simulink model "Study_1"  (R2023b)
settings: Solver=ode23s  StartTime=0.0  StopTime=150  RelTol=1e-3
values from neighbouring files (symbols this model uses):
  B = 1    [Study_1_data.m]
  K = 1    [Study_1_data.m]
  Kg = 0.8    [Study_1_data.m]
  M = 1    [Study_1_data.m]
  s = tf('s')    [Study_1_data.m]
libraries: slctrl_linear x15, simulink x6
settings Model: Creator=user  LastModifiedBy=user
settings SolverCC: AlgebraicLoopSolver=TrustRegion
settings DebuggingCC: UnconnectedInputMsg=warning  UnconnectedOutputMsg=warning  UnconnectedLineMsg=warning
settings ModelReferenceCC: EnableRefExpFcnMdlSchedulingChecks=on
settings RTWCC: DLArmComputeVersion=19.05

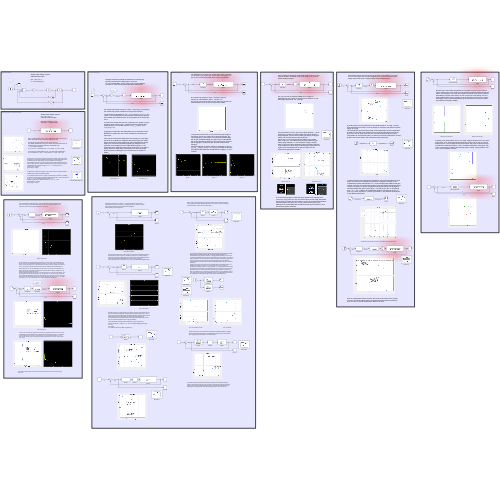
[thumbnail: Simulink's stored preview of the top-level diagram]
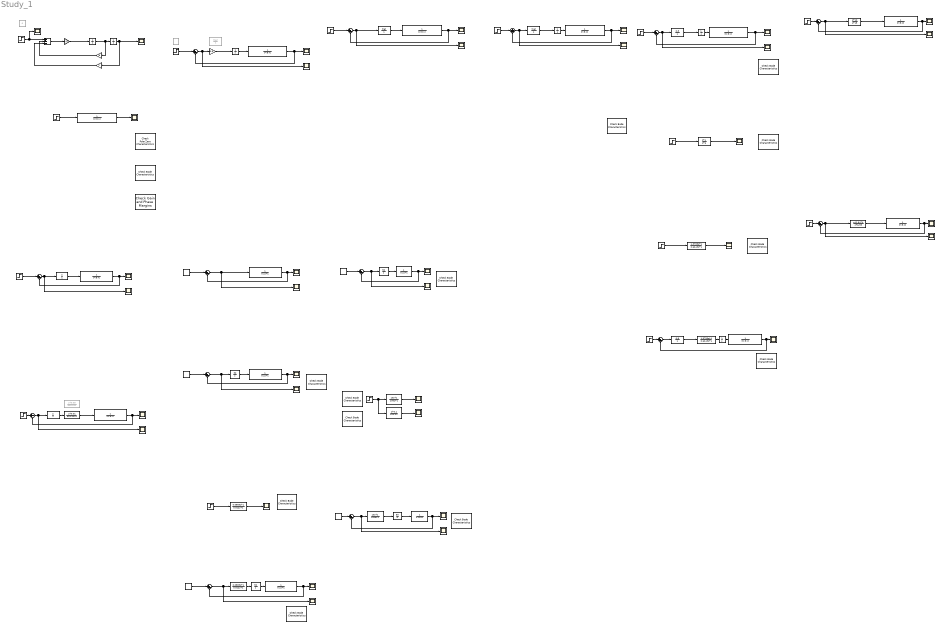
== system Study_1 ==
  note: Root Locus Study
  note: Closed loop System
  note: Basic Analysis for 2nd order system
  note: Differential Model
  note: @ Kg = 1
  note: Further more, we can plot our system response for frequency spectrum using
      | bode plots, by previous knowlegde we know that a second order system acts
      | as a filter due to its inertial nature, this is illustrated in the bode plot.
      | Quick bode plot preview, our second order system causes a decrease in gain after certain frequency, called the cutoff frequency, phase and gain margin are caulcated also from a bode plot, @ m = b = k = 1, cutoff freq at w = 1,
      | phase margin = 90 deg
      | gain margin = infinity.
  note: This is a second order system, using suitable calculations we can get certain parameters from it (rise time, settling time, etc)
      |
      | first lets get the pole locations for the open loop plant:
      | from simple calculations for this plant, there are 2 poles which have an imaginary part, the poles are found by characteristic eqn : (-b+- root(b^2-4ac))/2a
      | for m = b = k = 1, poles are at s1 = -0.5 + 0.86j , s2 = -0.5 - 0.86j
      |
      | we can find our natural frequency wn , and zeta from standard form
      | s^2 + 2*zeta*wn*s + wn^2 , in our case wn = 1 rad/s , zeta = 0.5
  note: Simple mass damper system
      | differential Eq model
      |
      | mx'' + bx' + kx = f
      | x'' = (F-kx-bx')(1/m)
  note: Simple mass damper system
      | mx'' + bx' + kx = F
      | Transfer function model
      |
      | (ms^2+bs+k)*X(s) = F(s)
      | X(s)/F(s) = 1/(ms^2+bs+k)
  note: studying closed loop systems is essential for controlling our plant and choosing the suitable type of controller.
      | For our demonstration, we are going to use a unity feedback controller, ie. Ideal sensing with no transient charactertics.
  note: the closed loop transfer function is: Gcl(s) = G(s)*Gc(s)/(1+G(s)Gc(s))
      | this closed loop system is stable from the previous analysis.
      |
      | The final value is calculated by, lim s->0 (1/s) *s*Gcl(s) = (1)/(1+1) = 0.5 ,where 1/s is the step input, s is from the final value theorem, and Gcl is the closed loop transfer function, so this system has an overall gain of 0.5
      |
      | to observe the steady state error for a step input, our system is a type 0 system, while a step is type 1, meaning that there will be a finite steady state error, to calculate the error -> lim s->0 s.R(s)/1+G(s) = 1/(1+(1/1)) = 0.5
  note: to assess our closed loop behavior even more we can do a nyquist plot to find stability margins and overall stability status.
      |
      | in our default example we have 2 open loop poles which 0 of them is unstable, and from the plot we have 0 clockwise rotations around the -1 point, from the rule: Z = N + P , -> the unstable closed loop poles are 0.
      | Stability margins for the default numbers of m = b = k = 1, are:
      | Phase margin = 90 deg
      | Gain margin = infinity
  note: by applying a ramp input, the steady state error is infinity due to the difference in system type, this can be illustrated by connecting the ramp input.
      |
      | if we want to eliminate the steady state error entirely for a step input, we can do so by adding an integrator (pole at the origin) this makes the input type equal to the system type, which eliminates the steady state error, this can be illustrated by adding an integrator block,
      | (note that: if the integrator block is added while the gain is 1, the system becomes marginally stable, which doesnt allow us to see the steady state error elimination, for illustration, we removed the Kg block and put a constant gain of 0.5 to make sure the system is stable.)
  note: Lets study the root locus for our closed loop system, assuming our controller is just a gain, lets see the effect of changing our gain on our closed loop system poles location and stability.
  note: Our closed loop system is: Gcl(s) = K*G(s)/(1+G(s)*K)
      | therefore our characteristic eqn is: 1+G(s)*K = 0,
      | lets plot our root locus for this c/cs eqn, this can't be done from inside simulink but we can do this from within matlab
  note: From the shown root locus we can see that the gain margin is sure infinite, and for our system as we increase the gain, the natural frequency of the system is increased and the damping ratio is also increased making the system more underdamped, this can be illustrated by observing the system's step response after changing the controller's gain, also the steady state is changing.
      | A general approach for steady state error assuming the gain is Kg, lim s->0 s.R(s)/(1+G(s)) = 1/(1+(Kg/1)), therefore we see that increasing Kg decreases the steady state error (@Kg = 5, Ess = 0.16667)
  note: @ Kg = 5
  note: @ Kg = 30
  note: Lets try adding an integrator to eliminate steady state error, then observe the effect of adding a pole at the origin on our overall system stability margins.
  note: Our c/cs eqn has an integrator added so we expect an additional pole, the number of asymptotes increases to 3, and their angles become 60, -60, 180 deg.
  note: From the shown root locus, we can see that if the gain > 1, then we become unstable, the system totally changed by adding a single integrator, it went from an infinite gain margin to tiny gain margin, we can illustrate this using bode plots.
      | Put our Kg = 0.5, this causes the gain margin to be 6.02db which is gain of 2, this makes sense since the maximum gain before going unstable is 1, also the phase margin is 50 deg which is fine as the larger the phase margin the faster response of the system, this can be seen by observing the settling time for a gain of 0.5 and settling time for gain of 0.8 (this can be achieved using stepinfo in matlab)
  note: Bode for Kg = 0.5
  note: Output @ Kg = 0.5
  note: Error @ Kg = 0.5
  note: Bode for Kg = 0.8
  note: As we increased the gain to make the poles approach the imaginary axis even more, ie: Kg from 0.5 to 0.8, we notice that the phase margin decreased, meaning that the system became harder to control as the phase shift between input and output is too large, also, as the system comes closer to the imaginary axis, the damping ratio decreases and the system settles in more time and has greater overshoot
  note: Lets assume that the system we have is the worst case possible, a Kg value of 0.8, it has 2 poles very near the imaginary axis, and it has almost no gain margin (we put the Kg as 0.8 permanently in the controller block)
  note: by observing the current system we have a phase margin of 14.3 deg , Lets put some requirements to meet, in order to design out controller, lets assume a phase margin of 30 deg.
      | This requirement can be achieved using a lead compensator, a lead compensator is made of a zero and a pole where the zero comes at lower frequency than the pole, ie the zero is closer to the real axis, this causes the bode plot of a lead compensator to have positive phase, so when we put a lead compensator, we add phase to the current system, this is illustrates using a bode plot.
  note: In order to find the lead compensator parameters, we should calculate how much phase we need, for our example we need about 16 degrees of phase, so our compensator's phase shift should be 16 + 6 (the 6 degrees are added as the gain shift will cause the zero-crossover frequency to be also shifted reducing the phase margin once again), to get the compensator equation that achieves 22 degrees maximum phase shift, get a (for 22 deg a = 2.2) and tao (for Wm =1.08 rad/s @ gain = -3.4 , tao = 0.6243), the compensator equation becomes ((a*tao*s)+1)/((tao*s)+1) which equates to (1.3735s+1)/(0.6243s+1), lets observe the bode plot of the added compensator.
  note: Another way to use a lead compensator is if we want to move our root locus to meet a certain point on the s plane, this is possible because by adding a pole and a zero, and the pole is to the left, this causes the centroid of the loci to be shifted left making the system more stable, we can control how much shifting occurs to meet a specific pole location, allowing us to get accurate results from our system, the shifting in the loci is illustrated below (for this illustration we used the system G(s) without an integrator added)
  note: Without lead compensator
  note: With lead compensator
  note: Currently our 2 poles location are at -0.5+-0.86j, suppose we want our lous to pass by the point -2+2j, using the angle argument (for a point to be on the loic, sum of angles of poles - sum of angles of zeros must equal 180), from the below analysis we find that to meet this condition, 145+113+thetaPole-thetaZero must equal 180, I chose a zero angle of 100deg, then the pole angle is 22deg, using geometry: zero is at -1.6474, and pole is at-6.95
  note: Compensator adds 22 deg at frequency of 0.88rad/s and also adds 3.43 db
  note: And our compensator doesnt work-ish, this is due to the nature of the system we have, its critically stable that any small gain increase causes our phase to drop so much, so a lead compensator doesn't work here.
  note: If our system has a steady state error, a lag compensator can be designed to limit that error using the root locus method, assume we have the system below, it has a SS error of 0.33 using a gain controller with value of 2.
  note: from the equation Z/P = (Gd(0)-Ess*Gd(0))/(Ess.Gn(0)), we can choose our desired Ess and get the ratio for our lag compensator transfer function, where Z is the location of the zero and P is the location of the pole, noting that for a lag compensator, the pole corner freq is always lower than the zero, so on the s-plane the pole will be to the left of the zero (opposite to a lead compensator).
      |
      | Assume an Ess of 0.1, then by substituting in the eqn: Z/P = 4.5, to create our compensator, we need to choose the zero position, First thing to know, we dont want to affect our original loci in the s-plane we just want to eliminate SS error.
      | The angle argument theorem tells us that for a point to fall on the loci, the sum of pole angles - sum of zero angles to that point must equal 180, so to not affect this loci, the pole and zero must be as close to each other as possible, so to the far right near the orgin, a good rule of thumb is to take the zero location as the Re(Dominant pole)/50, for our example our dominant pole is at s = -0.5+ 0.86j, so the zero is at s = -0.01, and the pole is at s=-0.0022, lets add our compensator.
  note: Before compensator
  note: From the root locus and error graphs we can see that our compensator works, the root locus and our dominant poles aren't affected, and the steady state error decreases to reach 0.1, the problem is that the reponse time is too slow, it takes about 10 mins to reach the desired error, so if we move the pole and zero a bit to the left the repsonse should be faster (let zero be -0.05 and pole be at -0.011)
  note: After compensator
  note: The response time got faster as the zero and pole were shifted to the left, but the rootlocus got bent more.
  note: Lets assume a plant of tf = 1/(0.2s+1) -> first order system, we have some requirements to meet in this system, a steady state error of less than 0.02 for ramp input and phase margin of greater than 48 degrees.
      | Lets first study our existing system.
  note: From analysis and from the existing graph, we can see that the steady state error is infinite, as the system type is 0, and the input type is 2, by adding a pole at origin to the system the steady state error can be finite, and by adding a gain we can choose our desired steady state error, Ess = R(s)/(1+(KG(s))).
      | so we calculate our K to be 50 for an error of 0.02, so we add an integrator (50/s)
  note: Error before Integrator
  note: Error after Integrator
  note: Now lets move to our phase margin reuqirements, from the bode plot we can see that we have about 18 degrees of phase margin and infinite gain margin, so we have a requirement of adding about 30 degrees of phase, this requirement can be achieved using a lead compensator, but also a lag compensator, a lag compensator can be used to solve both requirements at the same time, we will first use a lead compensator then the lag compensator.
      |
      | using calculations to design lead compensator: (a*tao*s+1)/(tao*s+1)
      | assume we add 30 + 7 degrees = 37 , W = 22 rad after adding gain1/root(a)
      | a = 4.02
      | tao = 0.022
      | our equation becomes (0.0885+1)/(0.022*s+1)
  note: We can use a lag compensator to achieve the phase margin required, he idea is that by shifting the whole magnitude plot down, we move the crossover frequency to lower frequency giving us more phase margin,
  note: by looking at the bode plot we see that to achieve a phase margin of 48 we need to shift the plot by subtracting about 18.5 db lets approximate to 20db, for a compensator to give gain shift of 20db, -> 20log(k)=20db, therefore k=10, then our compensator equation becomes (tao*s+1)/(beta*tao*s+1) where beta is 10, unlike a lead compensator we don't need to care about the phase shift of this compensator or at what frequency it's put, simply we choose a low frequency to not affect the dominant poles, and make sure the shift is totally applied before the zero crossover frequency.
      | a good rule of thumb is to choose the zero location at the dominantpole/50, in our equation this is Szero= -5/50 = -0.1, then the pole is at -0.1/10 = 0.01, our compensator equation becomes: (10*s+1)/(100*s+1) , note that the equation should be written like this because we are subtracting gain from 0 (at low freq s=jw=0, eqn evaluates to gain of 1 while at high freq s=jw=inf, eqn evaluates to 1/10,but if we write our equation as (s+0.1)/(s+0.01)), at low freq s=jw=0, eqn evaluates to gain of 1/10, while at freq s=jw=inf, eqn evaluates to gain of 1, we want the first case since we subtract gain from the total system, this is further illustrated below)
  note: This is the behavior we want
  note: This is undesired
  note: We can see that our compensator decreases gain by 20db and applies a negative phase shift of about 55deg at freq of 0.032rad/s, this should also be visible below when applying the compensator on the whole system.
  note: As we can see from the plot above the phase margin was increased to 50.5deg, and the gain crossover frequency was moved to 4 rad/s (previous analysis showed that the new crossover freq would be 4.43 rad/s), the spike at 0.0306 rad is due to applying the lag compensator which decreases phase at a chosen frequency
  Add : Sum  Inputs=+--
  Bode Plot : slctrl_linear/Check Bode  Characteristics  InstantiateOnLoad=on  SaveOperatingPoints=off  LinearizationIOs={'/Step1', 1, 'in', 'on', '';'/Transfer Fcn', 1, 'out', 'on', ''}  LinearizeAt=SnapshotTimes  SnapshotTimes=[0]  TriggerType=rising  SampleTime=auto  RateConversionMethod=zoh  PreWarpFreq=10  UseExactDelayModel=off  UseFullBlockNameLabels=off  UseBusSignalLabels=off  enabled=on  stopWhenAssertionFail=off  export=off  ViewDlgPos=[930 96 816 609]  OpenViewOnLoad=off  LaunchViewOnOpen=on  FrequencyUnits=rad/s  MagnitudeUnits=dB  PhaseUnits=deg  TimeUnits=seconds  EnableUpperBound=off  UpperBoundFrequencies=[]  UpperBoundMagnitudes=[]  EnableLowerBound=off  LowerBoundFrequencies=[]  LowerBoundMagnitudes=[]
      settings: SaveToWorkspace=off  SaveName=sys
  Bode Plot1 : slctrl_linear/Check Bode  Characteristics  InstantiateOnLoad=on  SaveOperatingPoints=off  LinearizationIOs={'/Sum2', 1, 'in', 'on', '';'/Plant2', 1, 'out', 'on', ''}  LinearizeAt=SnapshotTimes  SnapshotTimes=[0]  TriggerType=rising  SampleTime=auto  RateConversionMethod=zoh  PreWarpFreq=10  UseExactDelayModel=off  UseFullBlockNameLabels=off  UseBusSignalLabels=off  enabled=on  stopWhenAssertionFail=off  export=off  ViewDlgPos=[674 113 760 628]  OpenViewOnLoad=off  LaunchViewOnOpen=on  FrequencyUnits=rad/s  MagnitudeUnits=dB  PhaseUnits=deg  TimeUnits=seconds  EnableUpperBound=off  UpperBoundFrequencies=[]  UpperBoundMagnitudes=[]  EnableLowerBound=off  LowerBoundFrequencies=[]  LowerBoundMagnitudes=[]
      settings: SaveToWorkspace=off  SaveName=sys
  Bode Plot10 : slctrl_linear/Check Bode  Characteristics  InstantiateOnLoad=on  SaveOperatingPoints=off  LinearizationIOs={'/Step14', 1, 'in', 'on', '';'/Plant18', 1, 'out', 'on', ''}  LinearizeAt=SnapshotTimes  SnapshotTimes=[0]  TriggerType=rising  SampleTime=auto  RateConversionMethod=zoh  PreWarpFreq=10  UseExactDelayModel=off  UseFullBlockNameLabels=off  UseBusSignalLabels=off  enabled=on  stopWhenAssertionFail=off  export=off  ViewDlgPos=[197 143.4 656.8 567.2]  OpenViewOnLoad=off  LaunchViewOnOpen=on  FrequencyUnits=rad/s  MagnitudeUnits=dB  PhaseUnits=deg  TimeUnits=seconds  EnableUpperBound=off  UpperBoundFrequencies=[]  UpperBoundMagnitudes=[]  EnableLowerBound=off  LowerBoundFrequencies=[]  LowerBoundMagnitudes=[]
      settings: SaveToWorkspace=off  SaveName=sys
  Bode Plot11 : slctrl_linear/Check Bode  Characteristics  InstantiateOnLoad=on  SaveOperatingPoints=off  LinearizationIOs={'/Step14', 1, 'in', 'on', '';'/Plant19', 1, 'out', 'on', ''}  LinearizeAt=SnapshotTimes  SnapshotTimes=[0]  TriggerType=rising  SampleTime=auto  RateConversionMethod=zoh  PreWarpFreq=10  UseExactDelayModel=off  UseFullBlockNameLabels=off  UseBusSignalLabels=off  enabled=on  stopWhenAssertionFail=off  export=off  ViewDlgPos=[100 90.6 574.6 499.4]  OpenViewOnLoad=off  LaunchViewOnOpen=on  FrequencyUnits=rad/s  MagnitudeUnits=dB  PhaseUnits=deg  TimeUnits=seconds  EnableUpperBound=off  UpperBoundFrequencies=[]  UpperBoundMagnitudes=[]  EnableLowerBound=off  LowerBoundFrequencies=[]  LowerBoundMagnitudes=[]
      settings: SaveToWorkspace=off  SaveName=sys
  Bode Plot12 : slctrl_linear/Check Bode  Characteristics  InstantiateOnLoad=on  SaveOperatingPoints=off  LinearizationIOs={'/Sum13', 1, 'in', 'on', '';'/Plant21', 1, 'out', 'on', ''}  LinearizeAt=SnapshotTimes  SnapshotTimes=[0]  TriggerType=rising  SampleTime=auto  RateConversionMethod=zoh  PreWarpFreq=10  UseExactDelayModel=off  UseFullBlockNameLabels=off  UseBusSignalLabels=off  enabled=on  stopWhenAssertionFail=off  export=off  ViewDlgPos=[397 108.2 843.2 632.8]  OpenViewOnLoad=off  LaunchViewOnOpen=on  FrequencyUnits=rad/s  MagnitudeUnits=dB  PhaseUnits=deg  TimeUnits=seconds  EnableUpperBound=off  UpperBoundFrequencies=[]  UpperBoundMagnitudes=[]  EnableLowerBound=off  LowerBoundFrequencies=[]  LowerBoundMagnitudes=[]
      settings: SaveToWorkspace=off  SaveName=sys
  Bode Plot2 : slctrl_linear/Check Bode  Characteristics  InstantiateOnLoad=on  SaveOperatingPoints=off  LinearizationIOs={'/Sum3', 1, 'in', 'on', '';'/Plant3', 1, 'out', 'on', ''}  LinearizeAt=SnapshotTimes  SnapshotTimes=[0]  TriggerType=rising  SampleTime=auto  RateConversionMethod=zoh  PreWarpFreq=10  UseExactDelayModel=off  UseFullBlockNameLabels=off  UseBusSignalLabels=off  enabled=on  stopWhenAssertionFail=off  export=off  ViewDlgPos=[249 49 973.6 733.6]  OpenViewOnLoad=off  LaunchViewOnOpen=on  FrequencyUnits=rad/s  MagnitudeUnits=dB  PhaseUnits=deg  TimeUnits=seconds  EnableUpperBound=off  UpperBoundFrequencies=[]  UpperBoundMagnitudes=[]  EnableLowerBound=off  LowerBoundFrequencies=[]  LowerBoundMagnitudes=[]
      settings: SaveToWorkspace=off  SaveName=sys
  Bode Plot3 : slctrl_linear/Check Bode  Characteristics  InstantiateOnLoad=on  SaveOperatingPoints=off  LinearizationIOs={'/Transfer Fcn1', 1, 'out', 'on', '';'/Step9', 1, 'in', 'on', ''}  LinearizeAt=SnapshotTimes  SnapshotTimes=[0]  TriggerType=rising  SampleTime=auto  RateConversionMethod=zoh  PreWarpFreq=10  UseExactDelayModel=off  UseFullBlockNameLabels=off  UseBusSignalLabels=off  enabled=on  stopWhenAssertionFail=off  export=off  ViewDlgPos=[579 70 798 661]  OpenViewOnLoad=off  LaunchViewOnOpen=on  FrequencyUnits=rad/s  MagnitudeUnits=dB  PhaseUnits=deg  TimeUnits=seconds  EnableUpperBound=off  UpperBoundFrequencies=[]  UpperBoundMagnitudes=[]  EnableLowerBound=off  LowerBoundFrequencies=[]  LowerBoundMagnitudes=[]
      settings: SaveToWorkspace=off  SaveName=sys
  Bode Plot4 : slctrl_linear/Check Bode  Characteristics  InstantiateOnLoad=on  SaveOperatingPoints=off  LinearizationIOs={'/Sum4', 1, 'in', 'on', '';'/Plant4', 1, 'out', 'on', ''}  LinearizeAt=SnapshotTimes  SnapshotTimes=[0]  TriggerType=rising  SampleTime=auto  RateConversionMethod=zoh  PreWarpFreq=10  UseExactDelayModel=off  UseFullBlockNameLabels=off  UseBusSignalLabels=off  enabled=on  stopWhenAssertionFail=off  export=off  ViewDlgPos=[296.2 -8.6 940.8 791.2]  OpenViewOnLoad=off  LaunchViewOnOpen=on  FrequencyUnits=rad/s  MagnitudeUnits=dB  PhaseUnits=deg  TimeUnits=seconds  EnableUpperBound=off  UpperBoundFrequencies=[]  UpperBoundMagnitudes=[]  EnableLowerBound=off  LowerBoundFrequencies=[]  LowerBoundMagnitudes=[]
      settings: SaveToWorkspace=off  SaveName=sys
  Bode Plot5 : slctrl_linear/Check Bode  Characteristics  InstantiateOnLoad=on  SaveOperatingPoints=off  LinearizationIOs={'/Step10', 1, 'in', 'on', '';'/Transfer Fcn4', 1, 'out', 'on', ''}  LinearizeAt=SnapshotTimes  SnapshotTimes=[0]  TriggerType=rising  SampleTime=auto  RateConversionMethod=zoh  PreWarpFreq=10  UseExactDelayModel=off  UseFullBlockNameLabels=off  UseBusSignalLabels=off  enabled=on  stopWhenAssertionFail=off  export=off  ViewDlgPos=[1 1 799.2 595.2]  OpenViewOnLoad=off  LaunchViewOnOpen=on  FrequencyUnits=rad/s  MagnitudeUnits=dB  PhaseUnits=deg  TimeUnits=seconds  EnableUpperBound=off  UpperBoundFrequencies=[]  UpperBoundMagnitudes=[]  EnableLowerBound=off  LowerBoundFrequencies=[]  LowerBoundMagnitudes=[]
      settings: SaveToWorkspace=off  SaveName=sys
  Bode Plot6 : slctrl_linear/Check Bode  Characteristics  InstantiateOnLoad=on  SaveOperatingPoints=off  LinearizationIOs={'/Sum10', 1, 'in', 'on', '';'/Plant10', 1, 'out', 'on', ''}  LinearizeAt=SnapshotTimes  SnapshotTimes=[0]  TriggerType=rising  SampleTime=auto  RateConversionMethod=zoh  PreWarpFreq=10  UseExactDelayModel=off  UseFullBlockNameLabels=off  UseBusSignalLabels=off  enabled=on  stopWhenAssertionFail=off  export=off  ViewDlgPos=[805.8 114.6 677.6 612]  OpenViewOnLoad=off  LaunchViewOnOpen=on  FrequencyUnits=rad/s  MagnitudeUnits=dB  PhaseUnits=deg  TimeUnits=seconds  EnableUpperBound=off  UpperBoundFrequencies=[]  UpperBoundMagnitudes=[]  EnableLowerBound=off  LowerBoundFrequencies=[]  LowerBoundMagnitudes=[]
      settings: SaveToWorkspace=off  SaveName=sys
  Bode Plot7 : slctrl_linear/Check Bode  Characteristics  InstantiateOnLoad=on  SaveOperatingPoints=off  LinearizationIOs={'/Sum11', 1, 'in', 'on', '';'/Plant12', 1, 'out', 'on', ''}  LinearizeAt=SnapshotTimes  SnapshotTimes=[0]  TriggerType=rising  SampleTime=auto  RateConversionMethod=zoh  PreWarpFreq=10  UseExactDelayModel=off  UseFullBlockNameLabels=off  UseBusSignalLabels=off  enabled=on  stopWhenAssertionFail=off  export=off  ViewDlgPos=[96.2 122.6 704.8 616.8]  OpenViewOnLoad=off  LaunchViewOnOpen=on  FrequencyUnits=rad/s  MagnitudeUnits=dB  PhaseUnits=deg  TimeUnits=seconds  EnableUpperBound=off  UpperBoundFrequencies=[]  UpperBoundMagnitudes=[]  EnableLowerBound=off  LowerBoundFrequencies=[]  LowerBoundMagnitudes=[]
      settings: SaveToWorkspace=off  SaveName=sys
  Bode Plot8 : slctrl_linear/Check Bode  Characteristics  InstantiateOnLoad=on  SaveOperatingPoints=off  LinearizationIOs={'/Step13', 1, 'in', 'on', '';'/Plant15', 1, 'out', 'on', ''}  LinearizeAt=SnapshotTimes  SnapshotTimes=[0]  TriggerType=rising  SampleTime=auto  RateConversionMethod=zoh  PreWarpFreq=10  UseExactDelayModel=off  UseFullBlockNameLabels=off  UseBusSignalLabels=off  enabled=on  stopWhenAssertionFail=off  export=off  ViewDlgPos=[250.6 79.4 677.6 607.2]  OpenViewOnLoad=off  LaunchViewOnOpen=on  FrequencyUnits=rad/s  MagnitudeUnits=dB  PhaseUnits=deg  TimeUnits=seconds  EnableUpperBound=off  UpperBoundFrequencies=[]  UpperBoundMagnitudes=[]  EnableLowerBound=off  LowerBoundFrequencies=[]  LowerBoundMagnitudes=[]
      settings: SaveToWorkspace=off  SaveName=sys
  Bode Plot9 : slctrl_linear/Check Bode  Characteristics  InstantiateOnLoad=on  SaveOperatingPoints=off  LinearizationIOs={'/Sum10', 1, 'in', 'on', '';'/Plant10', 1, 'out', 'on', ''}  LinearizeAt=SnapshotTimes  SnapshotTimes=[0]  TriggerType=rising  SampleTime=auto  RateConversionMethod=zoh  PreWarpFreq=10  UseExactDelayModel=off  UseFullBlockNameLabels=off  UseBusSignalLabels=off  enabled=on  stopWhenAssertionFail=off  export=off  ViewDlgPos=[397.8 97.8 743.2 606.4]  OpenViewOnLoad=off  LaunchViewOnOpen=on  FrequencyUnits=rad/s  MagnitudeUnits=dB  PhaseUnits=deg  TimeUnits=seconds  EnableUpperBound=off  UpperBoundFrequencies=[]  UpperBoundMagnitudes=[]  EnableLowerBound=off  LowerBoundFrequencies=[]  LowerBoundMagnitudes=[]
      settings: SaveToWorkspace=off  SaveName=sys
  Constant : Constant  Commented=on  Value=0
  Controller : TransferFcn  Commented=on  Numerator=[Kg]  Denominator=[1]
  Controller1 : TransferFcn  Numerator=[Kg]  Denominator=[1]
  Controller2 : TransferFcn  Numerator=[Kg]  Denominator=[1]
  Controller3 : TransferFcn  Numerator=[0.8]  Denominator=[1]
  Controller4 : TransferFcn  Numerator=[0.8]  Denominator=[1]
  Controller5 : TransferFcn  Numerator=[2]  Denominator=[1]
  Controller6 : TransferFcn  Numerator=[2]  Denominator=[1]
  Controller7 : TransferFcn  Commented=on  Numerator=[1 0.05]  Denominator=[1 0.011]
  Controller8 : TransferFcn  Numerator=[1 0.01]  Denominator=[1 0.0022]
  Error{,1..14} (15 alike) : Scope
  Gain : Gain  Gain=K
  Gain and Phase Margin Plot : slctrl_linear/Check Gain and Phase Margins  InstantiateOnLoad=on  SaveOperatingPoints=off  LinearizationIOs={'/Step1', 1, 'in', 'on', '';'/Transfer Fcn', 1, 'out', 'on', ''}  LinearizeAt=SnapshotTimes  SnapshotTimes=[0]  TriggerType=rising  SampleTime=auto  RateConversionMethod=zoh  PreWarpFreq=10  UseExactDelayModel=off  UseFullBlockNameLabels=off  UseBusSignalLabels=off  enabled=on  stopWhenAssertionFail=off  export=off  ViewDlgPos=[946 210 635 570]  LaunchViewOnOpen=on  OpenViewOnLoad=off  FrequencyUnits=rad/s  MagnitudeUnits=dB  PhaseUnits=deg  TimeUnits=seconds  EnableMargins=off  GainMargin=[]  PhaseMargin=[]  PlotType=nyquist  FeedbackSign=-1
      settings: SaveToWorkspace=off  SaveName=sys
  Gain1 : Gain  Gain=B
  Gain2 : Gain  Gain=1/M
  Gain3 : Gain  Gain=0.5
  Integrator{,1..5} (6 alike) : Integrator
  Lead Compensator : TransferFcn  Numerator=[1 10]  Denominator=[1 15]
  Lead Compensator1 : TransferFcn  Numerator=[1 1.6474]  Denominator=[1 6.95]
  Plant{,1..8} (9 alike) : TransferFcn  Denominator=[M B K]
  Plant{9..10,12,16,21} (5 alike) : TransferFcn  Denominator=[0.2 1]
  Plant{11,13,17,22} (4 alike) : TransferFcn  Numerator=[50]  Denominator=[1 0]
  Plant14 : TransferFcn  Numerator=[0.0885 1]  Denominator=[0.022 1]
  Plant15 : TransferFcn  Numerator=[0.0885 1]  Denominator=[0.022 1]
  Plant18 : TransferFcn  Numerator=[10 1]  Denominator=[100 1]
  Plant19 : TransferFcn  Numerator=[1 0.1]  Denominator=[1 0.01]
  Plant20 : TransferFcn  Numerator=[10 1]  Denominator=[100 1]
  Pole-Zero Plot : slctrl_linear/Check Pole-Zero Characteristics  InstantiateOnLoad=on  SaveOperatingPoints=off  LinearizationIOs={'/Step1', 1, 'in', 'on', '';'/Transfer Fcn', 1, 'out', 'on', ''}  LinearizeAt=SnapshotTimes  SnapshotTimes=[0]  TriggerType=rising  SampleTime=auto  RateConversionMethod=zoh  PreWarpFreq=10  UseExactDelayModel=off  UseFullBlockNameLabels=off  UseBusSignalLabels=off  enabled=on  stopWhenAssertionFail=off  export=off  ViewDlgPos=[658 159 890 670]  LaunchViewOnOpen=on  OpenViewOnLoad=off  FrequencyUnits=rad/s  MagnitudeUnits=dB  PhaseUnits=deg  TimeUnits=seconds  EnableSettlingTime=off  SettlingTime=[]  EnablePercentOvershoot=off  PercentOvershoot=[]  EnableDampingRatio=off  DampingRatio=[]  EnableNaturalFrequency=off  NaturalFrequencyBound=>=  NaturalFrequency=[]
      settings: SaveToWorkspace=off  SaveName=sys
  Ramp : simulink/Sources/Ramp  Commented=on  slope=1  start=0  InitialOutput=0
  Ramp{1..5} (5 alike) : simulink/Sources/Ramp  slope=1  start=0  InitialOutput=0
  Scope{,1..19} (20 alike) : Scope
  Step : Step  SampleTime=0
  Step{1..12} (12 alike) : Step  Time=0  SampleTime=0
  Step13 : Step  SampleTime=0
  Step14 : Step  SampleTime=0
  Sum{,1..13} (14 alike) : Sum  Inputs=|+-
  Transfer Fcn : TransferFcn  Denominator=[M B K]
  Transfer Fcn1 : TransferFcn  Numerator=[1 4]  Denominator=[1 6]
  Transfer Fcn2 : TransferFcn  Numerator=[1.3735 1]  Denominator=[0.6243 1]
  Transfer Fcn4 : TransferFcn  Numerator=[1.3735 1]  Denominator=[0.6243 1]
  wires:
  Integrator1/1 -> Gain/1, Scope/1  "x"
  Integrator/1 -> Gain1/1, Integrator1/1  "x'"
  Gain2/1 -> Integrator/1  "x''"
  Gain/1 -> Add/3  "Kx"
  Gain1/1 -> Add/2  "Bx'"
  Step/1 -> Scope11/1, Add/1  "f"
  Add/1 -> Gain2/1  "x''"
  Step1/1 -> Transfer Fcn/1  "F"
  Transfer Fcn/1 -> Scope1/1  "x"
  Plant/1 -> Scope2/1, Sum/2  "x"
  Sum/1 -> Gain3/1, Error/1  "Error"
  Step2/1 -> Sum/1  "F"
  Gain3/1 -> Integrator4/1  "Actuation"
  Controller1/1 -> Plant1/1  "Actuation"
  Step3/1 -> Sum1/1  "F"
  Sum1/1 -> Controller1/1, Error1/1  "Error"
  Plant1/1 -> Sum1/2, Scope3/1  "x"
  Plant2/1 -> Scope4/1, Sum2/2  "x"
  Sum2/1 -> Error2/1, Controller2/1  "Error"
  Step4/1 -> Sum2/1  "F"
  Controller2/1 -> Integrator3/1  "Actuation"
  Integrator3/1 -> Plant2/1
  Integrator4/1 -> Plant/1
  Integrator2/1 -> Plant3/1
  Controller3/1 -> Integrator2/1  "Actuation"
  Step5/1 -> Sum3/1  "F"
  Sum3/1 -> Controller3/1, Error3/1  "Error"
  Plant3/1 -> Sum3/2, Scope5/1  "x"
  Plant4/1 -> Scope6/1, Sum4/2  "x"
  Sum4/1 -> Controller4/1  "Error"
  Step6/1 -> Sum4/1  "F"
  Controller4/1 -> Transfer Fcn2/1  "Actuation"
  Integrator5/1 -> Plant4/1
  Transfer Fcn2/1 -> Integrator5/1
  Step7/1 -> Sum5/1  "F"
  Sum5/1 -> Lead Compensator/1, Error5/1
  Plant5/1 -> Sum5/2, Scope7/1  "x"
  Lead Compensator/1 -> Plant5/1
  Lead Compensator1/1 -> Plant6/1
  Plant6/1 -> Scope8/1, Sum6/2  "x"
  Sum6/1 -> Error6/1, Lead Compensator1/1  "Error"
  Step8/1 -> Sum6/1  "F"
  Step9/1 -> Transfer Fcn1/1  "Compensator in"
  Transfer Fcn1/1 -> Error7/1  "Compensator out"
  Transfer Fcn4/1 -> Error8/1  "Compensator out"
  Step10/1 -> Transfer Fcn4/1  "Compensator in"
  Plant7/1 -> Sum7/2, Scope12/1  "x"
  Sum7/1 -> Error4/1, Controller5/1  "Error"
  Step11/1 -> Sum7/1  "F"
  Controller5/1 -> Plant7/1  "Actuation"
  Controller6/1 -> Controller8/1
  Step12/1 -> Sum8/1  "F"
  Sum8/1 -> Controller6/1, Error9/1  "Error"
  Plant8/1 -> Scope13/1, Sum8/2  "x"
  Controller8/1 -> Plant8/1  "Actuation"
  Sum9/1 -> Plant9/1, Error10/1  "Error"
  Ramp2/1 -> Sum9/1  "F"
  Plant9/1 -> Scope14/1, Sum9/2  "x"
  Plant10/1 -> Sum10/2, Scope15/1  "x"
  Ramp3/1 -> Sum10/1  "F"
  Sum10/1 -> Error11/1, Plant11/1  "Error"
  Plant11/1 -> Plant10/1  "x"
  Plant13/1 -> Plant12/1  "x"
  Sum11/1 -> Plant14/1, Error12/1  "Error"
  Ramp4/1 -> Sum11/1  "F"
  Plant12/1 -> Scope16/1, Sum11/2  "x"
  Plant14/1 -> Plant13/1  "x"
  Plant15/1 -> Scope17/1  "x"
  Step13/1 -> Plant15/1
  Plant17/1 -> Plant16/1  "x"
  Sum12/1 -> Plant17/1, Error13/1  "Error"
  Ramp1/1 -> Sum12/1  "F"
  Plant16/1 -> Scope9/1, Sum12/2  "x"
  Step14/1 -> Plant19/1, Plant18/1
  Plant18/1 -> Scope10/1  "x"
  Plant19/1 -> Scope18/1  "x"
  Ramp5/1 -> Sum13/1  "F"
  Sum13/1 -> Error14/1, Plant20/1  "Error"
  Plant20/1 -> Plant22/1  "x"
  Plant22/1 -> Plant21/1  "x"
  Plant21/1 -> Scope19/1, Sum13/2  "x"
